simulink model "untitled"  (R2025a)
settings: Solver=VariableStepAuto  StartTime=0.0  StopTime=10.0  RelTol=1e-3
InitFcn:
  | run('LongitudinalABS.m')
values from neighbouring files (symbols this model uses):
  Fz_const = mq*g    (= 3678.75)    [LongitudinalABS.m]
  J = 1.2    [LongitudinalABS.m]
  lambda_high = 0.18    [LongitudinalABS.m]
  lambda_low = 0.12    [LongitudinalABS.m]
  mq = m/4    (= 375)    [LongitudinalABS.m]
  omega0 = v0/R    (= 92.6)    [LongitudinalABS.m]
  R = 0.30    (= 0.3)    [LongitudinalABS.m]
  Tb_max = 3000    [LongitudinalABS.m]
  Tb_rate_dn = -6000    [LongitudinalABS.m]
  Tb_rate_up = 1500    [LongitudinalABS.m]
  v0 = 27.78    [LongitudinalABS.m]
  v_abs_off = 1.0    (= 1)    [LongitudinalABS.m]
  v_eps = 0.5    [LongitudinalABS.m]
undefined symbols (not defined in the file or in its folder): Road
libraries: simulink x3
settings Model: Creator=muhan  LastModifiedBy=muhan

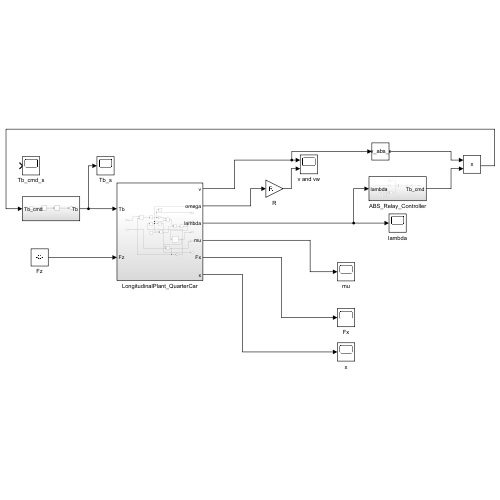
[thumbnail: Simulink's stored preview of the top-level diagram]
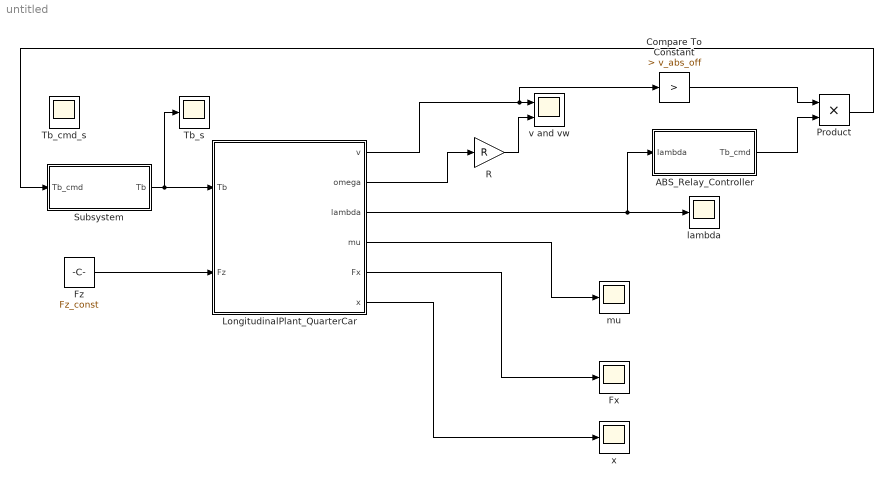
== system untitled ==
  ABS_Relay_Controller : Subsystem
  Compare To Constant : simulink/Logic and Bit Operations/Compare To Constant  relop=>  const=v_abs_off  OutDataTypeStr=boolean
  Fx : Scope
      settings: ActiveDisplayYMinimum=-458.29560675387569  ActiveDisplayYMaximum=4124.6604607848822  DataLoggingVariableName=ScopeData4
  Fz : Constant  Value=Fz_const
  LongitudinalPlant_QuarterCar : Subsystem
  Product : Product
  R : Gain  Gain=R
  Subsystem : Subsystem
  Tb_cmd_s : Scope
      settings: ActiveDisplayYMinimum=-252.92457113415344  ActiveDisplayYMaximum=2276.3211402073816
  Tb_s : Scope
      settings: ActiveDisplayYMinimum=-165.04181830405491  ActiveDisplayYMaximum=1485.3763647364945  DataLoggingVariableName=ScopeData7
  lambda : Scope
      settings: ActiveDisplayYMinimum=-0.022500000000000627  ActiveDisplayYMaximum=0.20250000000000568  DataLoggingVariableName=ScopeData2
  mu : Scope
      settings: ActiveDisplayYMinimum=0.01608422823678135  ActiveDisplayYMaximum=0.89055099512649949  DataLoggingVariableName=ScopeData3
  v and vw : Scope  NumInputPorts=2
      settings: ActiveDisplayYMinimum=-3.4724999999999993  ActiveDisplayYMaximum=31.2525
  x : Scope
      settings: ActiveDisplayYMinimum=-114.44328033287998  ActiveDisplayYMaximum=75.288306682730678  DataLoggingVariableName=ScopeData5
  wires:
  Fz/1 -> LongitudinalPlant_QuarterCar/2(Fz)
  LongitudinalPlant_QuarterCar/1(v) -> Compare To Constant/1, v and vw/1
  LongitudinalPlant_QuarterCar/2(omega) -> R/1
  R/1 -> v and vw/2
  LongitudinalPlant_QuarterCar/3(lambda) -> lambda/1, ABS_Relay_Controller/1(lambda)
  LongitudinalPlant_QuarterCar/4(mu) -> mu/1
  LongitudinalPlant_QuarterCar/5(Fx) -> Fx/1
  LongitudinalPlant_QuarterCar/6(x) -> x/1
  Subsystem/1(Tb) -> Tb_s/1, LongitudinalPlant_QuarterCar/1(Tb)
  Compare To Constant/1 -> Product/1
  ABS_Relay_Controller/1(Tb_cmd) -> Product/2
  Product/1 -> Subsystem/1(Tb_cmd)

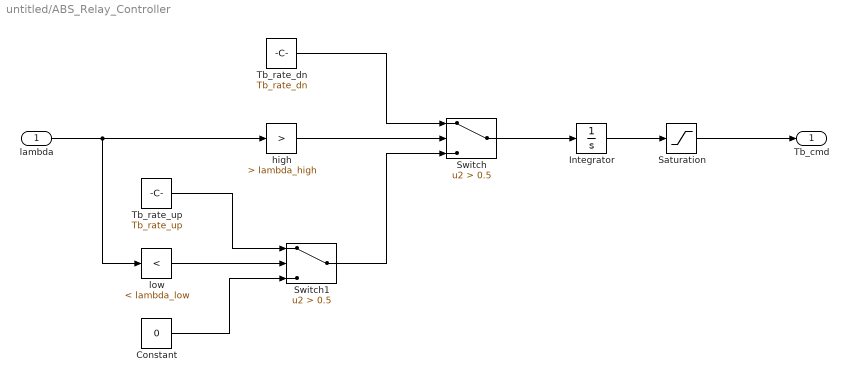
== system untitled/ABS_Relay_Controller ==
  lambda : Inport
  Constant : Constant  Value=0
  Integrator : Integrator
  Saturation : Saturate  UpperLimit=Tb_max  LowerLimit=0
  Switch : Switch  Criteria=u2 > Threshold  Threshold=0.5  SaturateOnIntegerOverflow=off  InputSameDT=off
  Switch1 : Switch  Criteria=u2 > Threshold  Threshold=0.5  SaturateOnIntegerOverflow=off  InputSameDT=off
  Tb_rate_dn : Constant  Value=Tb_rate_dn
  Tb_rate_up : Constant  Value=Tb_rate_up
  high : simulink/Logic and Bit Operations/Compare To Constant  relop=>  const=lambda_high  OutDataTypeStr=boolean
  low : simulink/Logic and Bit Operations/Compare To Constant  relop=<  const=lambda_low  OutDataTypeStr=boolean
  Tb_cmd : Outport
  wires:
  lambda/1 -> low/1, high/1
  high/1 -> Switch/2
  Tb_rate_dn/1 -> Switch/1
  Switch1/1 -> Switch/3
  low/1 -> Switch1/2
  Tb_rate_up/1 -> Switch1/1
  Constant/1 -> Switch1/3
  Switch/1 -> Integrator/1
  Integrator/1 -> Saturation/1
  Saturation/1 -> Tb_cmd/1

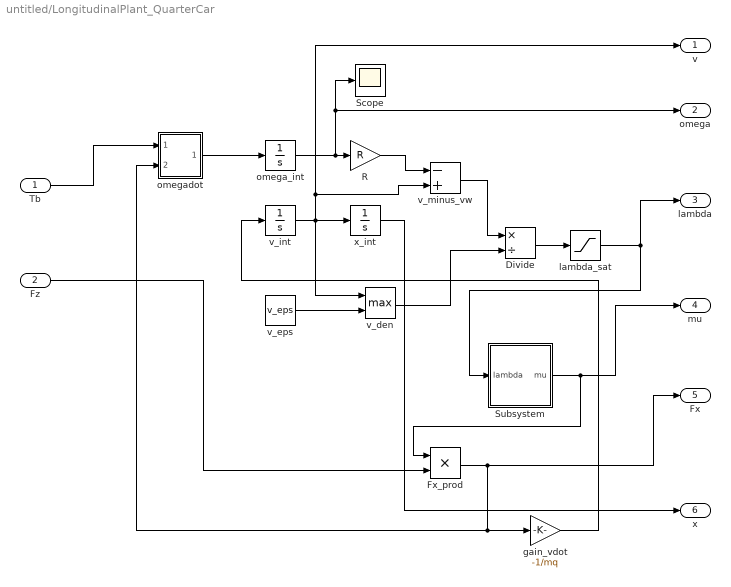
== system untitled/LongitudinalPlant_QuarterCar ==
  Tb : Inport
  Fz : Inport  Port=2
  Divide : Product  Inputs=*/
  Fx_prod : Product
  R : Gain  Gain=R
  Scope : Scope
      settings: ActiveDisplayYMinimum=-6.0492755786504944  ActiveDisplayYMaximum=104.1888196594448  DataLoggingVariableName=ScopeData6
  Subsystem : Subsystem
  gain_vdot : Gain  Gain=-1/mq
  lambda_sat : Saturate  UpperLimit=1  LowerLimit=0
  omega_int : Integrator  InitialCondition=omega0  LimitOutput=on  LowerSaturationLimit=0
  omegadot : Subsystem
  v_den : MinMax  Function=max  Inputs=2
  v_eps : Constant  Value=v_eps
  v_int : Integrator  InitialCondition=v0  LimitOutput=on  LowerSaturationLimit=0
  v_minus_vw : Sum  Inputs=-+
  x_int : Integrator
  v : Outport
  omega : Outport  Port=2
  lambda : Outport  Port=3
  mu : Outport  Port=4
  Fx : Outport  Port=5
  x : Outport  Port=6
  wires:
  v_int/1 -> v_minus_vw/2, v/1, v_den/1, x_int/1
  omega_int/1 -> omega/1, Scope/1, R/1
  v_eps/1 -> v_den/2
  R/1 -> v_minus_vw/1
  v_minus_vw/1 -> Divide/1
  v_den/1 -> Divide/2
  Divide/1 -> lambda_sat/1
  lambda_sat/1 -> Subsystem/1(lambda), lambda/1
  Subsystem/1(mu) -> Fx_prod/1, mu/1
  Fz/1 -> Fx_prod/2
  Fx_prod/1 -> Fx/1, gain_vdot/1, omegadot/2(In2)
  gain_vdot/1 -> v_int/1
  Tb/1 -> omegadot/1(In1)
  omegadot/1(Out1) -> omega_int/1
  x_int/1 -> x/1

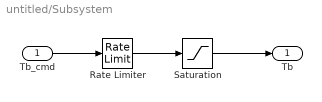
== system untitled/Subsystem ==
  Tb_cmd : Inport
  Rate Limiter : RateLimiter  RisingSlewLimit=Tb_rate_up  FallingSlewLimit=Tb_rate_dn  SampleTimeMode=inherited
  Saturation : Saturate  UpperLimit=Tb_max  LowerLimit=0
  Tb : Outport
  wires:
  Tb_cmd/1 -> Rate Limiter/1
  Rate Limiter/1 -> Saturation/1
  Saturation/1 -> Tb/1

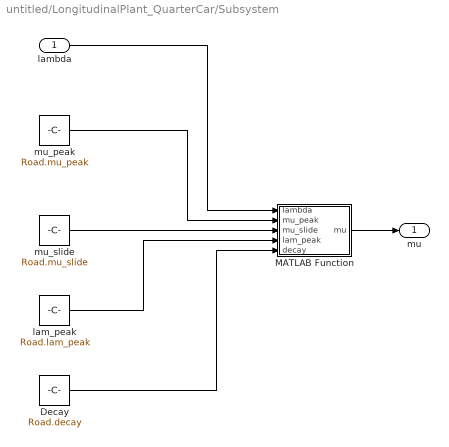
== system untitled/LongitudinalPlant_QuarterCar/Subsystem ==
  lambda : Inport
  Decay : Constant  Value=Road.decay
  MATLAB Function : MATLAB Function  TreatAsAtomicUnit=on
  lam_peak : Constant  Value=Road.lam_peak
  mu_peak : Constant  Value=Road.mu_peak
  mu_slide : Constant  Value=Road.mu_slide
  mu : Outport
  wires:
  lambda/1 -> MATLAB Function/1(lambda)
  mu_peak/1 -> MATLAB Function/2(mu_peak)
  mu_slide/1 -> MATLAB Function/3(mu_slide)
  Decay/1 -> MATLAB Function/5(decay)
  lam_peak/1 -> MATLAB Function/4(lam_peak)
  MATLAB Function/1(mu) -> mu/1

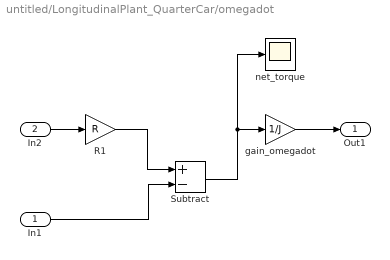
== system untitled/LongitudinalPlant_QuarterCar/omegadot ==
  In1 : Inport
  In2 : Inport  Port=2
  R1 : Gain  Gain=R
  Subtract : Sum  Inputs=+-
  gain_omegadot : Gain  Gain=1/J
  net_torque : Scope
      settings: ActiveDisplayYMinimum=-1  ActiveDisplayYMaximum=1  DataLoggingVariableName=ScopeData21
  Out1 : Outport
  wires:
  gain_omegadot/1 -> Out1/1
  In1/1 -> Subtract/2
  R1/1 -> Subtract/1
  Subtract/1 -> net_torque/1, gain_omegadot/1
  In2/1 -> R1/1

== matlab function untitled/LongitudinalPlant_QuarterCar/Subsystem/MATLAB Function ==
  data: lambda input; mu output; mu_peak input; mu_slide input; lam_peak input; decay input
function mu = TireMu(lambda, mu_peak, mu_slide, lam_peak, decay)
% TireMu: simple physically-plausible mu(slip) curve for braking
% lambda   : slip ratio in [0..1]
% mu_peak  : peak friction coefficient
% mu_slide : sliding friction coefficient at high slip
% lam_peak : slip at peak friction (~0.1-0.2 dry)
% decay    : decay shaping parameter (>0)

% clamp inputs (defensive)
if lambda < 0
    lambda = 0;
elseif lambda > 1
    lambda = 1;
end

if lam_peak <= 0
    lam_peak = 0.15;
end
if decay <= 0
    decay = 0.10;
end

% piecewise curve: rise to peak, then decay to sliding level
if lambda <= lam_peak
    mu = mu_peak * (lambda / lam_peak);
else
    mu = mu_slide + (mu_peak - mu_slide) * exp(-(lambda - lam_peak)/decay);
end

% final clamp (just in case)
if mu < 0
    mu = 0;
end
end
